simulink model "Final_integration_correctoin_after"  (R2023b)
settings: Solver=FixedStepAuto  StartTime=0.0  StopTime=inf  FixedStep=Ts  RelTol=1e-3
InitFcn:
  | params
  | pin_params
undefined symbols (not defined in the file or in its folder): b, default1, den_Gd, encoder_scale, f, J, Kb, KD, Kf, KI, Km, KP, l, L, num_Gd, r, R, steering, Vlim, Wref
libraries: arduinolib x27, simulink x6, arduinosensorlib x6
(part 2 of 2)

== system Final_integration_correctoin_after/Subsystem4/Subsystem/If Action Subsystem11/If Action Subsystem1 ==
  In1 : Inport
  In2 : Inport  Port=2
  Action Port : ActionPort
  Constant : Constant  Value=0
  If : If  NumInputs=2  IfExpression=(u1<10)&(u2<10)  ElseIfExpressions=u1<10,u2<10
  If Action Subsystem : Subsystem  TreatAsAtomicUnit=on
  If Action Subsystem1 : Subsystem  TreatAsAtomicUnit=on
  If Action Subsystem2 : Subsystem  TreatAsAtomicUnit=on
  If Action Subsystem3 : Subsystem  TreatAsAtomicUnit=on
  Merge : Merge  Inputs=4
  Merge1 : Merge  Inputs=4
  Out1 : Outport
  Out2 : Outport  Port=2
  Out3 : Outport  Port=3
  wires:
  In1/1 -> If Action Subsystem1/1(In3), If Action Subsystem/1(In3), If/1
  If/1 -> If Action Subsystem/Action
  In2/1 -> If Action Subsystem2/1(In3), If Action Subsystem/2(In4), If/2
  If/2 -> If Action Subsystem1/Action
  If/3 -> If Action Subsystem2/Action
  If/4 -> If Action Subsystem3/Action
  If Action Subsystem/1(Out1) -> Merge/1
  If Action Subsystem1/1(Out2) -> Merge/2
  If Action Subsystem2/1(Out2) -> Merge/3
  If Action Subsystem3/1(Out1) -> Merge/4
  If Action Subsystem/2(Out2) -> Merge1/1
  If Action Subsystem1/2(Out3) -> Merge1/2
  If Action Subsystem2/2(Out3) -> Merge1/3
  If Action Subsystem3/2(Out2) -> Merge1/4
  Merge/1 -> Out1/1
  Merge1/1 -> Out2/1
  Constant/1 -> Out3/1

== system Final_integration_correctoin_after/Subsystem4/Subsystem/If Action Subsystem11/If Action Subsystem2 ==
  In1 : Inport
  In2 : Inport  Port=2
  Action Port : ActionPort
  Out1 : Outport
  Out2 : Outport  Port=2
  wires:
  In1/1 -> Out1/1
  In2/1 -> Out2/1

== system Final_integration_correctoin_after/Subsystem4/Subsystem/If Action Subsystem11/If Action Subsystem3 ==
  In1 : Inport
  In2 : Inport  Port=2
  Action Port : ActionPort
  Gain : Gain  Gain=1.2
  Gain1 : Gain  Gain=1.2
  Out1 : Outport
  Out2 : Outport  Port=2
  wires:
  In1/1 -> Gain/1
  Gain/1 -> Out1/1
  In2/1 -> Gain1/1
  Gain1/1 -> Out2/1

== system Final_integration_correctoin_after/Subsystem4/Subsystem/If Action Subsystem3/If Action Subsystem ==
  Action Port : ActionPort
  Constant : Constant  Value=0
  Constant1 : Constant  Value=0
  Out1 : Outport
  Out2 : Outport  Port=2
  wires:
  Constant1/1 -> Out2/1
  Constant/1 -> Out1/1

== system Final_integration_correctoin_after/Subsystem4/Subsystem/If Action Subsystem3/If Action Subsystem1 ==
  In1 : Inport
  In2 : Inport  Port=2
  Action Port : ActionPort
  If : If  NumInputs=2  IfExpression=(u1<10)&(u2<10)  ElseIfExpressions=u1<10,u2<10
  If Action Subsystem : Subsystem  TreatAsAtomicUnit=on
  If Action Subsystem1 : Subsystem  TreatAsAtomicUnit=on
  If Action Subsystem2 : Subsystem  TreatAsAtomicUnit=on
  If Action Subsystem3 : Subsystem  TreatAsAtomicUnit=on
  Merge : Merge  Inputs=4
  Merge1 : Merge  Inputs=4
  Out1 : Outport
  Out2 : Outport  Port=2
  wires:
  In1/1 -> If Action Subsystem1/1(In3), If Action Subsystem/1(In3), If/1
  If/1 -> If Action Subsystem/Action
  In2/1 -> If Action Subsystem2/1(In3), If Action Subsystem/2(In4), If/2
  If/2 -> If Action Subsystem1/Action
  If/3 -> If Action Subsystem2/Action
  If/4 -> If Action Subsystem3/Action
  If Action Subsystem/1(Out1) -> Merge/1
  If Action Subsystem1/1(Out2) -> Merge/2
  If Action Subsystem2/1(Out2) -> Merge/3
  If Action Subsystem3/1(Out1) -> Merge/4
  If Action Subsystem/2(Out2) -> Merge1/1
  If Action Subsystem1/2(Out3) -> Merge1/2
  If Action Subsystem2/2(Out3) -> Merge1/3
  If Action Subsystem3/2(Out2) -> Merge1/4
  Merge/1 -> Out1/1
  Merge1/1 -> Out2/1

== system Final_integration_correctoin_after/Subsystem4/Subsystem/If Action Subsystem3/If Action Subsystem2 ==
  In1 : Inport
  In2 : Inport  Port=2
  Action Port : ActionPort
  Out1 : Outport
  Out2 : Outport  Port=2
  wires:
  In1/1 -> Out1/1
  In2/1 -> Out2/1

== system Final_integration_correctoin_after/Subsystem4/Subsystem/If Action Subsystem3/If Action Subsystem3 ==
  In1 : Inport
  In2 : Inport  Port=2
  Action Port : ActionPort
  Gain : Gain  Gain=1.2
  Gain1 : Gain  Gain=1.2
  Out1 : Outport
  Out2 : Outport  Port=2
  wires:
  In1/1 -> Gain/1
  Gain/1 -> Out1/1
  In2/1 -> Gain1/1
  Gain1/1 -> Out2/1

== system Final_integration_correctoin_after/light_Ctrl/Subsystem/Subsystem/If Action Subsystem ==
  In1 : Inport
  Action Port : ActionPort  ActionPortLabel=if(u1 == 0)
  Out1 : Outport
  Out2 : Outport  Port=2
  wires:
  In1/1 -> Out2/1, Out1/1

== system Final_integration_correctoin_after/light_Ctrl/Subsystem/Subsystem/If Action Subsystem1 ==
  light : Inport
  In1 : Inport  Port=2
  Action Port : ActionPort  ActionPortLabel=elseif(u1 == 1)
  Constant : Constant
  Constant1 : Constant  Value=0
  If : If  IfExpression=u1 <= 150
  If Action Subsystem : Subsystem  TreatAsAtomicUnit=on
  If Action Subsystem1 : Subsystem  TreatAsAtomicUnit=on
  Merge : Merge
  Out1 : Outport
  Out2 : Outport  Port=2
  wires:
  light/1 -> If/1
  Constant/1 -> If Action Subsystem/1(In1)
  Constant1/1 -> If Action Subsystem1/1(In1)
  If/1 -> If Action Subsystem/Action
  If/2 -> If Action Subsystem1/Action
  If Action Subsystem/1(Out1) -> Merge/1
  If Action Subsystem1/1(Out1) -> Merge/2
  Merge/1 -> Out1/1
  In1/1 -> Out2/1

== system Final_integration_correctoin_after/light_Ctrl/Subsystem/Subsystem/If Action Subsystem2 ==
  In1 : Inport
  Action Port : ActionPort  ActionPortLabel=elseif( u1 == 2)
  Out1 : Outport
  Out2 : Outport  Port=2
  wires:
  In1/1 -> Out2/1, Out1/1

== system Final_integration_correctoin_after/State_Ctrl/drive_mode/SW1/If Action Subsystem1/If Action Subsystem ==
  In1 : Inport
  Action Port : ActionPort  ActionPortLabel=else
  Out1 : Outport
  wires:
  In1/1 -> Out1/1

== system Final_integration_correctoin_after/State_Ctrl/drive_mode/SW1/If Action Subsystem1/If Action Subsystem1 ==
  In1 : Inport
  Action Port : ActionPort  ActionPortLabel=if((u1 == 0) & (u2 == 0) )
  Out1 : Outport
  wires:
  In1/1 -> Out1/1

== system Final_integration_correctoin_after/Subsystem4/Subsystem/If Action Subsystem11/If Action Subsystem1/If Action Subsystem ==
  In3 : Inport
  In4 : Inport  Port=2
  Action Port : ActionPort
  Constant : Constant  Value=default1
  Constant1 : Constant  Value=steering
  Constant2 : Constant
  Constant3 : Constant  Value=default1
  Product : Product
  Product1 : Product
  Product3 : Product
  Subtract : Sum  Inputs=+-
  Subtract1 : Sum  Inputs=+-
  Subtract3 : Sum
  Out1 : Outport
  Out2 : Outport  Port=2
  wires:
  Subtract/1 -> Product/2
  Constant1/1 -> Product/1
  Subtract1/1 -> Product1/2
  Product/1 -> Subtract1/2, Subtract3/2
  Constant/1 -> Product1/1
  Product1/1 -> Out1/1
  Subtract3/1 -> Product3/2
  Constant2/1 -> Subtract3/1, Subtract1/1
  In4/1 -> Subtract/2
  Constant3/1 -> Product3/1
  In3/1 -> Subtract/1
  Product3/1 -> Out2/1

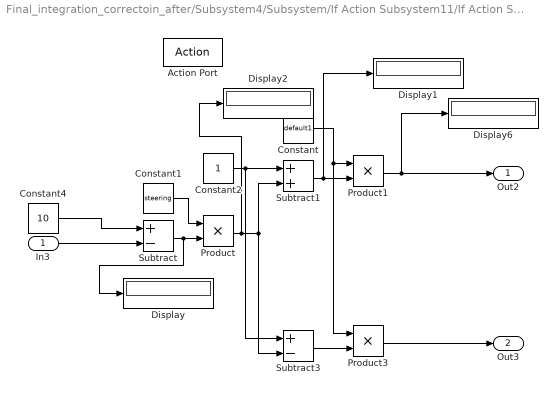
== system Final_integration_correctoin_after/Subsystem4/Subsystem/If Action Subsystem11/If Action Subsystem1/If Action Subsystem1 ==
  In3 : Inport
  Action Port : ActionPort
  Constant : Constant  Value=default1
  Constant1 : Constant  Value=steering
  Constant2 : Constant
  Constant4 : Constant  Value=10
  Display{,1..2,6} (4 alike) : Display
  Product : Product  OutDataTypeStr=double  RndMeth=Convergent
  Product1 : Product  OutDataTypeStr=double  RndMeth=Convergent
  Product3 : Product  OutDataTypeStr=double  RndMeth=Convergent
  Subtract : Sum  Inputs=+-  OutDataTypeStr=double  RndMeth=Convergent
  Subtract1 : Sum  OutDataTypeStr=double  RndMeth=Convergent
  Subtract3 : Sum  Inputs=+-  OutDataTypeStr=double  RndMeth=Convergent
  Out2 : Outport
  Out3 : Outport  Port=2
  wires:
  Product/1 -> Display2/1, Subtract1/2, Subtract3/2
  Subtract1/1 -> Display1/1, Product1/2
  Constant1/1 -> Product/1
  Constant2/1 -> Subtract3/1, Subtract1/1
  In3/1 -> Subtract/2
  Subtract/1 -> Display/1, Product/2
  Subtract3/1 -> Product3/2
  Product3/1 -> Out3/1
  Constant/1 -> Product3/1, Product1/1
  Product1/1 -> Display6/1, Out2/1
  Constant4/1 -> Subtract/1

== system Final_integration_correctoin_after/Subsystem4/Subsystem/If Action Subsystem11/If Action Subsystem1/If Action Subsystem2 ==
  In3 : Inport
  Action Port : ActionPort
  Constant : Constant  Value=default1
  Constant1 : Constant  Value=steering
  Constant2 : Constant
  Constant4 : Constant  Value=10
  Product : Product
  Product1 : Product
  Product3 : Product
  Subtract : Sum  Inputs=+-
  Subtract1 : Sum  Inputs=+-
  Subtract3 : Sum
  Out2 : Outport
  Out3 : Outport  Port=2
  wires:
  Constant4/1 -> Subtract/1
  Constant/1 -> Product3/1, Product1/1
  Product/1 -> Subtract1/2, Subtract3/2
  Product3/1 -> Out3/1
  Subtract3/1 -> Product3/2
  Subtract/1 -> Product/2
  Subtract1/1 -> Product1/2
  Product1/1 -> Out2/1
  Constant1/1 -> Product/1
  Constant2/1 -> Subtract3/1, Subtract1/1
  In3/1 -> Subtract/2

== system Final_integration_correctoin_after/Subsystem4/Subsystem/If Action Subsystem11/If Action Subsystem1/If Action Subsystem3 ==
  Action Port : ActionPort
  Constant : Constant  Value=360
  Constant1 : Constant  Value=360
  Out1 : Outport
  Out2 : Outport  Port=2
  wires:
  Constant/1 -> Out1/1
  Constant1/1 -> Out2/1

== system Final_integration_correctoin_after/Subsystem4/Subsystem/If Action Subsystem3/If Action Subsystem1/If Action Subsystem ==
  In3 : Inport
  In4 : Inport  Port=2
  Action Port : ActionPort
  Constant : Constant  Value=default1
  Constant1 : Constant  Value=steering
  Constant2 : Constant
  Constant3 : Constant  Value=default1
  Product : Product
  Product1 : Product
  Product3 : Product
  Subtract : Sum  Inputs=+-
  Subtract1 : Sum  Inputs=+-
  Subtract3 : Sum
  Out1 : Outport
  Out2 : Outport  Port=2
  wires:
  Subtract/1 -> Product/2
  Constant1/1 -> Product/1
  Subtract1/1 -> Product1/2
  Product/1 -> Subtract1/2, Subtract3/2
  Constant/1 -> Product1/1
  Product1/1 -> Out1/1
  Subtract3/1 -> Product3/2
  Constant2/1 -> Subtract3/1, Subtract1/1
  In4/1 -> Subtract/2
  Constant3/1 -> Product3/1
  In3/1 -> Subtract/1
  Product3/1 -> Out2/1

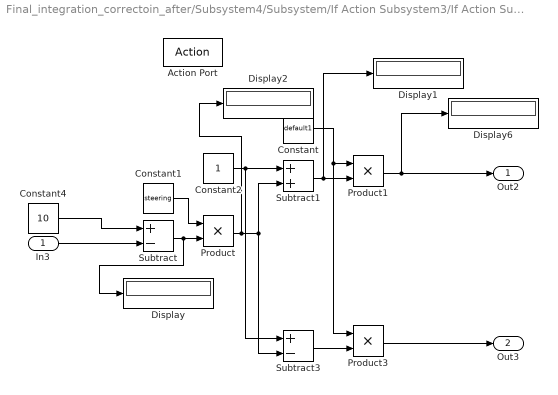
== system Final_integration_correctoin_after/Subsystem4/Subsystem/If Action Subsystem3/If Action Subsystem1/If Action Subsystem1 ==
  In3 : Inport
  Action Port : ActionPort
  Constant : Constant  Value=default1
  Constant1 : Constant  Value=steering
  Constant2 : Constant
  Constant4 : Constant  Value=10
  Display{,1..2,6} (4 alike) : Display
  Product : Product  OutDataTypeStr=double  RndMeth=Convergent
  Product1 : Product  OutDataTypeStr=double  RndMeth=Convergent
  Product3 : Product  OutDataTypeStr=double  RndMeth=Convergent
  Subtract : Sum  Inputs=+-  OutDataTypeStr=double  RndMeth=Convergent
  Subtract1 : Sum  OutDataTypeStr=double  RndMeth=Convergent
  Subtract3 : Sum  Inputs=+-  OutDataTypeStr=double  RndMeth=Convergent
  Out2 : Outport
  Out3 : Outport  Port=2
  wires:
  Product/1 -> Display2/1, Subtract1/2, Subtract3/2
  Subtract1/1 -> Display1/1, Product1/2
  Constant1/1 -> Product/1
  Constant2/1 -> Subtract3/1, Subtract1/1
  In3/1 -> Subtract/2
  Subtract/1 -> Display/1, Product/2
  Subtract3/1 -> Product3/2
  Product3/1 -> Out3/1
  Constant/1 -> Product3/1, Product1/1
  Product1/1 -> Display6/1, Out2/1
  Constant4/1 -> Subtract/1

== system Final_integration_correctoin_after/Subsystem4/Subsystem/If Action Subsystem3/If Action Subsystem1/If Action Subsystem2 ==
  In3 : Inport
  Action Port : ActionPort
  Constant : Constant  Value=default1
  Constant1 : Constant  Value=steering
  Constant2 : Constant
  Constant4 : Constant  Value=10
  Product : Product
  Product1 : Product
  Product3 : Product
  Subtract : Sum  Inputs=+-
  Subtract1 : Sum  Inputs=+-
  Subtract3 : Sum
  Out2 : Outport
  Out3 : Outport  Port=2
  wires:
  Constant4/1 -> Subtract/1
  Constant/1 -> Product3/1, Product1/1
  Product/1 -> Subtract1/2, Subtract3/2
  Product3/1 -> Out3/1
  Subtract3/1 -> Product3/2
  Subtract/1 -> Product/2
  Subtract1/1 -> Product1/2
  Product1/1 -> Out2/1
  Constant1/1 -> Product/1
  Constant2/1 -> Subtract3/1, Subtract1/1
  In3/1 -> Subtract/2

== system Final_integration_correctoin_after/Subsystem4/Subsystem/If Action Subsystem3/If Action Subsystem1/If Action Subsystem3 ==
  Action Port : ActionPort
  Constant : Constant  Value=360
  Constant1 : Constant  Value=360
  Out1 : Outport
  Out2 : Outport  Port=2
  wires:
  Constant/1 -> Out1/1
  Constant1/1 -> Out2/1

== system Final_integration_correctoin_after/light_Ctrl/Subsystem/Subsystem/If Action Subsystem1/If Action Subsystem ==
  In1 : Inport
  Action Port : ActionPort  ActionPortLabel=if(u1 <= 150)
  Out1 : Outport
  wires:
  In1/1 -> Out1/1

== system Final_integration_correctoin_after/light_Ctrl/Subsystem/Subsystem/If Action Subsystem1/If Action Subsystem1 ==
  In1 : Inport
  Action Port : ActionPort  ActionPortLabel=else
  Out1 : Outport
  wires:
  In1/1 -> Out1/1

== stateflow chart Final_integration_correctoin_after/Chart ==
  state AccOff
    en: state=state+1;
    v1=sw1;
    v2=sw2;
    n=state/100
    du:
  state AccStandby
    en: state=state+1;
    v1=sw1;
    v2=sw2;
    n=state/100
    du:
  state AccOn1
    en: state=state-1;
    v1=sw1;
    v2=sw2;
    n=state/100
    du:
  state AccOn
    en: state=state-1;
    v1=sw1;
    v2=sw2;
    n=state/100
    du:
  (default) -> AccOff : {state=-1}
  AccOff -> AccStandby [order 1] : [v1~=sw1]
  AccStandby -> AccOff [order 1] : [v1~=sw1]
  AccOff -> AccOn [order 2] : [v2~=sw2]
  AccOn -> AccOff [order 2] : [v1~=sw1]
  AccOn1 -> AccStandby [order 1] : [v1~=sw1]
  AccStandby -> AccOn1 [order 2] : [v2~=sw2]
  AccOn1 -> AccOn [order 2] : [v2~=sw2]
  AccOn -> AccOn1 [order 1] : [v2~=sw2]
  data: sw1 input; v1 local; v2 local; sw2 input; n output; state local

== stateflow chart Final_integration_correctoin_after/light_Ctrl/Subsystem/Chart1 ==
  state light_auto
    en, du:
    light_mode = 1;
    state_1 = sw3;
  state light_off
    en, du:
    light_mode =0;
    state_1 = sw3;
  state light_on
    en,du:
    light_mode =2;
    state_1 = sw3;
  light_auto -> (junction 15) : [(state_1 ~= sw3) && (Drive_mode == 1)]
  (junction 12) -> light_auto
  (junction 15) -> light_on
  light_off -> (junction 12) : [(state_1 ~= sw3) && (Drive_mode == 1)]
  (default) -> light_off
  light_on -> light_off : [(state_1 ~= sw3) && (Drive_mode == 1)]
  data: sw3 input; Drive_mode input; state_1 local; light_mode output

== stateflow chart Final_integration_correctoin_after/Subsystem5/Chart1 ==
  state adas_off
    en,du:
    rout1=out1;
    rout2=out2;
  state adas_on
    en,du:
    rout1=out1;
    rout2=out2;
  state adas_on_BUS
    en,du:
    rout1=out1*1.2;
    rout2=out2*1.2;
  adas_on_BUS -> adas_off [order 2] : [adas_mode==0]
  (default) -> adas_off
  adas_on -> adas_on_BUS [order 2] : [BUS<=10]
  adas_off -> adas_on : [adas_mode==1]
  adas_on -> adas_off [order 1] : [adas_mode==0]
  adas_on_BUS -> adas_on [order 1] : [BUS>10]
  data: adas_mode input; out1 input; out2 input; BUS input; rout1 output; rout2 output

== stateflow chart Final_integration_correctoin_after/Subsystem5/Chart ==
  state drive_on_adas_on
    en, du:
    out1 = default;
    out2 = default;
  state drive_off
    en, du:
    out1 = 0;
    out2 = 0;
    steering = 0.02;
    default = 360;
  state drive_on_adas_off
    en, du:
    out1 = default*(1+(handle-128)/6.4/100);
    out2 = default*(1+(128-handle)/6.4/100);
    exit:
    buzzer = 0;
  state drive_on_adas_on_FUS
    en,du:
    out1 = 0;
    out2 = 0;
    buzzer = 1;
    exit:
    buzzer = 0;
  state drive_on_adas_on_LUS
    en,du:
    out1 = default*(1+(10-LUS)*steering);
    out2 = default*(1-(10-LUS)*steering);
  state drive_on_adas_on_RUS
    en,du:
    out1 = default*(1-(10-RUS)*steering);
    out2 = default*(1+(10-RUS)*steering);
  state drive_on_adas_on_LRUS
    en,du:
    out1 = default*(1-(LUS-RUS)*steering);
    out2 = default*(1+(LUS-RUS)*steering);
  drive_on_adas_on_FUS -> drive_on_adas_off [order 5] : [adas_mode ==0]
  (default) -> drive_off
  drive_on_adas_on -> drive_on_adas_on_FUS [order 2] : [FUS<=10]
  drive_on_adas_on_FUS -> drive_on_adas_on_LUS [order 4] : [LUS<=10&&FUS>10]
  drive_off -> drive_on_adas_off : [drive_mode==1]
  drive_on_adas_off -> drive_on_adas_on [order 2] : [adas_mode == 1]
  drive_on_adas_on_FUS -> drive_on_adas_on [order 1] : [LUS>10&&RUS>10&&FUS>10]
  drive_on_adas_off -> drive_off [order 1] : [drive_mode ==0]
  drive_on_adas_on_FUS -> drive_on_adas_on_LRUS [order 2] : [LUS<=10&&RUS<=10&&FUS>10]
  drive_on_adas_on -> drive_on_adas_off [order 1] : [adas_mode  == 0]
  drive_on_adas_on_RUS -> drive_on_adas_off [order 4] : [adas_mode ==0]
  drive_on_adas_on -> drive_on_adas_on_LUS [order 4] : [LUS<=10]
  drive_on_adas_on_LUS -> drive_on_adas_on [order 1] : [LUS>10]
  drive_on_adas_on -> drive_on_adas_on_RUS [order 3] : [RUS<=10]
  drive_on_adas_on_RUS -> drive_on_adas_on [order 1] : [RUS>10]
  drive_on_adas_on_LUS -> drive_on_adas_off [order 4] : [adas_mode ==0]
  drive_on_adas_on_LRUS -> drive_on_adas_off [order 4] : [adas_mode==0]
  drive_on_adas_on_LUS -> drive_on_adas_on_FUS [order 3] : [FUS<=10]
  drive_on_adas_on_LRUS -> drive_on_adas_on_FUS [order 1] : [FUS<=10]
  drive_on_adas_on_RUS -> drive_on_adas_on_FUS [order 2] : [FUS<=10]
  drive_on_adas_on_FUS -> drive_on_adas_on_RUS [order 3] : [RUS<=10&&FUS>10]
  drive_on_adas_on_RUS -> drive_on_adas_on_LRUS [order 3] : [LUS<=10]
  drive_on_adas_on_LRUS -> drive_on_adas_on_RUS [order 3] : [LUS>10]
  drive_on_adas_on_LUS -> drive_on_adas_on_LRUS [order 2] : [RUS<=10]
  drive_on_adas_on_LRUS -> drive_on_adas_on_LUS [order 2] : [RUS>10]
  data: drive_mode input; adas_mode input; FUS input; LUS input; RUS input; out1 output; out2 output; handle input double; buzzer output; steering local double; speed1 local double; speed2 local double; default local double
